simulink model "Linear_Bicycle_Model"  (R2020a)
settings: Solver=VariableStepAuto  StartTime=0.0  StopTime=10  RelTol=1e-3
values from neighbouring files (symbols this model uses):
  c_alpha_f = 156000    [init.m]
  c_alpha_r = 193000    [init.m]
  delta_max = deg2rad(37.3)    [init.m]
  Iz = 2937    [init.m]
  lf = 1.04    [init.m]
  lr = 1.40    (= 1.4)    [init.m]
  mass = 1919    [init.m]
  psi0 = 0*pi/180    (= 0)    [init.m]
  psid0 = 0    [init.m]
  steering_constant = deg2rad(10)    [init.m]
  steering_input_switch = 3    [init.m]
  steering_omega = 0.25    [init.m]
  steering_rate = deg2rad(2)    [init.m]
  v_lat0 = 0    [init.m]
  v_lon0 = 5    [init.m]
  x0 = 0    [init.m]
  y0 = -0.1    [init.m]
libraries: simulink x2
settings Model: Creator=Sameed Quais  LastModifiedBy=Sameed Quais

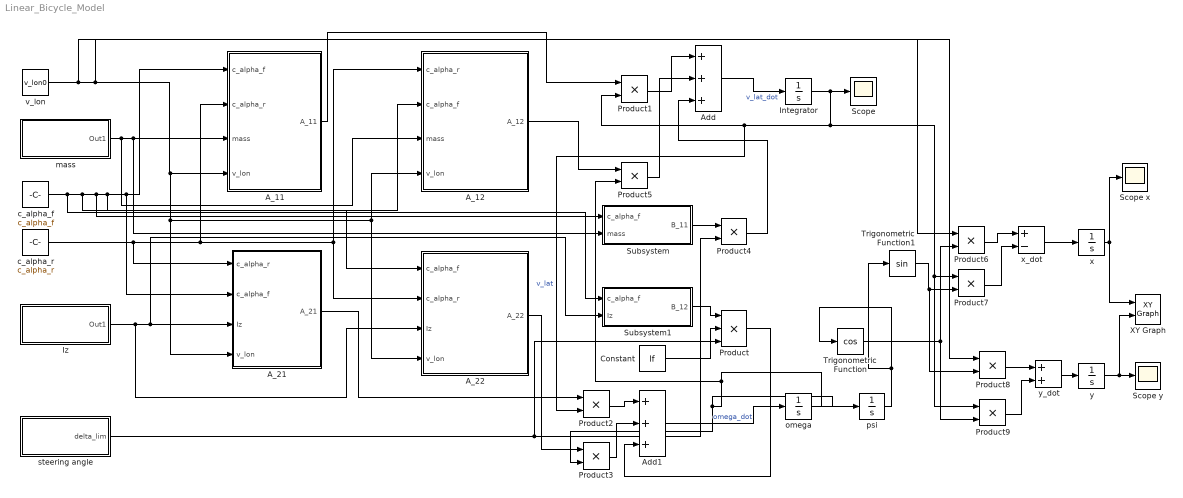
== system Linear_Bicycle_Model ==
  A_11 : Subsystem
  A_12 : Subsystem
  A_21 : Subsystem
  A_22 : Subsystem
  Add : Sum  Inputs=+++
  Add1 : Sum  Inputs=+++
  Constant : Constant  Value=lf
  Integrator : Integrator  InitialCondition=v_lat0
  Iz : Subsystem
  Product : Product  Inputs=3
  Product{1..9} (9 alike) : Product
  Scope : Scope
  Scope x : Scope
  Scope y : Scope
  Subsystem : Subsystem
  Subsystem1 : Subsystem
  Trigonometric Function : Trigonometry  Operator=cos
  Trigonometric Function1 : Trigonometry
  XY Graph : simulink/Sinks/XY Graph  xmin=-inf  xmax=inf  ymin=-inf  ymax=inf  st=-1
  c_alpha_f : Constant  Value=c_alpha_f
  c_alpha_r : Constant  Value=c_alpha_r
  mass : Subsystem
  omega : Integrator  InitialCondition=psi0
  psi : Integrator  InitialCondition=psid0
  steering angle : Subsystem
  v_lon : Constant  Value=v_lon0
  x : Integrator  InitialCondition=x0
  x_dot : Sum  Inputs=+-
  y : Integrator  InitialCondition=y0
  y_dot : Sum
  wires:
  Subsystem1/1(B_12) -> Product/1
  Constant/1 -> Product/2
  mass/1(Out1) -> A_12/3(mass), Subsystem/2(mass), A_11/3(mass)
  v_lon/1 -> Product6/1, Product8/1, A_22/4(v_lon), A_12/4(v_lon), A_21/4(v_lon), A_11/4(v_lon)
  c_alpha_f/1 -> Subsystem1/1(c_alpha_f), A_22/1(c_alpha_f), Subsystem/1(c_alpha_f), A_12/2(c_alpha_f), A_21/2(c_alpha_f), A_11/1(c_alpha_f)
  c_alpha_r/1 -> A_22/2(c_alpha_r), A_12/1(c_alpha_r), A_11/2(c_alpha_r), A_21/1(c_alpha_r)
  Iz/1(Out1) -> A_22/3(Iz), Subsystem1/2(Iz), A_21/3(Iz)
  A_11/1(A_11) -> Product1/1
  Integrator/1 -> Product9/1, Product7/1, Product2/2, Product1/2, Scope/1  "v_lat"
  A_21/1(A_21) -> Product2/1
  omega/1 -> Product3/2, psi/1, Product5/2
  A_22/1(A_22) -> Product3/1
  Subsystem/1(B_11) -> Product4/1
  steering angle/1(delta_lim) -> Product/3, Product4/2
  Product1/1 -> Add/1
  Add/1 -> Integrator/1  "v_lat_dot"
  A_12/1(A_12) -> Product5/1
  Product5/1 -> Add/2
  Product4/1 -> Add/3
  Product2/1 -> Add1/1
  Add1/1 -> omega/1  "omega_dot"
  Product/1 -> Add1/3
  Product3/1 -> Add1/2
  psi/1 -> Trigonometric Function1/1, Trigonometric Function/1
  Trigonometric Function/1 -> Product9/2, Product6/2
  Product6/1 -> x_dot/1
  Trigonometric Function1/1 -> Product8/2, Product7/2
  Product7/1 -> x_dot/2
  x_dot/1 -> x/1
  Product8/1 -> y_dot/1
  Product9/1 -> y_dot/2
  y_dot/1 -> y/1
  x/1 -> Scope x/1, XY Graph/1
  y/1 -> XY Graph/2, Scope y/1

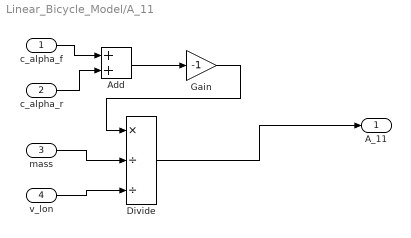
== system Linear_Bicycle_Model/A_11 ==
  c_alpha_f : Inport
  c_alpha_r : Inport  Port=2
  mass : Inport  Port=3
  v_lon : Inport  Port=4
  Add : Sum
  Divide : Product  Inputs=*//
  Gain : Gain  Gain=-1
  A_11 : Outport
  wires:
  c_alpha_r/1 -> Add/2
  c_alpha_f/1 -> Add/1
  mass/1 -> Divide/2
  v_lon/1 -> Divide/3
  Add/1 -> Gain/1
  Gain/1 -> Divide/1
  Divide/1 -> A_11/1

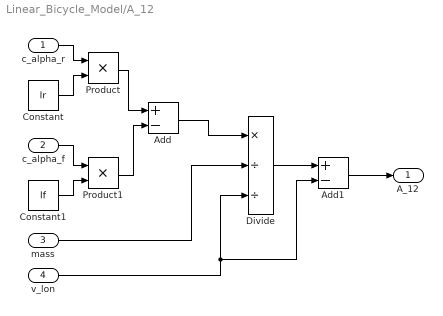
== system Linear_Bicycle_Model/A_12 ==
  c_alpha_r : Inport
  c_alpha_f : Inport  Port=2
  mass : Inport  Port=3
  v_lon : Inport  Port=4
  Add : Sum  Inputs=+-
  Add1 : Sum  Inputs=+-
  Constant : Constant  Value=lr
  Constant1 : Constant  Value=lf
  Divide : Product  Inputs=*//
  Product : Product
  Product1 : Product
  A_12 : Outport
  wires:
  c_alpha_r/1 -> Product/1
  Constant/1 -> Product/2
  c_alpha_f/1 -> Product1/1
  Constant1/1 -> Product1/2
  Product/1 -> Add/1
  Product1/1 -> Add/2
  Add/1 -> Divide/1
  mass/1 -> Divide/2
  v_lon/1 -> Add1/2, Divide/3
  Divide/1 -> Add1/1
  Add1/1 -> A_12/1

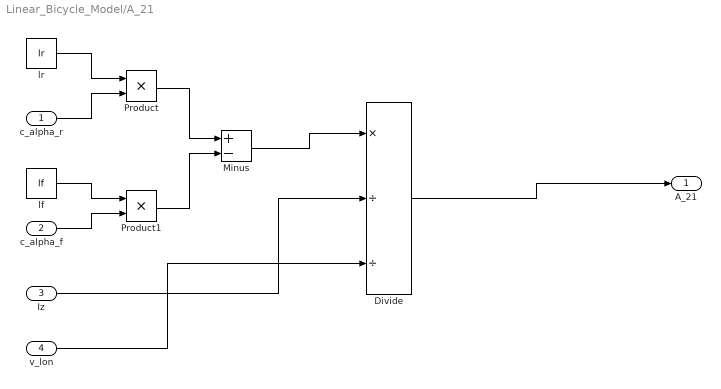
== system Linear_Bicycle_Model/A_21 ==
  c_alpha_r : Inport
  c_alpha_f : Inport  Port=2
  Iz : Inport  Port=3
  v_lon : Inport  Port=4
  Divide : Product  Inputs=*//
  Minus : Sum  Inputs=+-
  Product : Product
  Product1 : Product
  lf : Constant  Value=lf
  lr : Constant  Value=lr
  A_21 : Outport
  wires:
  lr/1 -> Product/1
  c_alpha_r/1 -> Product/2
  lf/1 -> Product1/1
  c_alpha_f/1 -> Product1/2
  Product/1 -> Minus/1
  Product1/1 -> Minus/2
  Minus/1 -> Divide/1
  Iz/1 -> Divide/2
  v_lon/1 -> Divide/3
  Divide/1 -> A_21/1

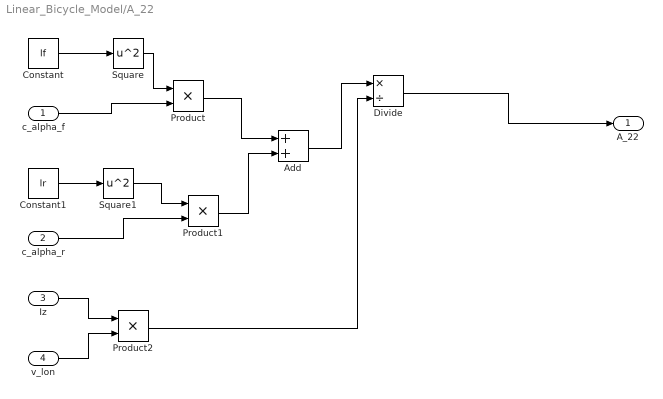
== system Linear_Bicycle_Model/A_22 ==
  c_alpha_f : Inport
  c_alpha_r : Inport  Port=2
  Iz : Inport  Port=3
  v_lon : Inport  Port=4
  Add : Sum
  Constant : Constant  Value=lf
  Constant1 : Constant  Value=lr
  Divide : Product  Inputs=*/
  Product : Product
  Product1 : Product
  Product2 : Product
  Square : Math  Operator=square  SaturateOnIntegerOverflow=on
  Square1 : Math  Operator=square  SaturateOnIntegerOverflow=on
  A_22 : Outport
  wires:
  Constant/1 -> Square/1
  Square/1 -> Product/1
  c_alpha_f/1 -> Product/2
  Constant1/1 -> Square1/1
  c_alpha_r/1 -> Product1/2
  Square1/1 -> Product1/1
  Product/1 -> Add/1
  Product1/1 -> Add/2
  Add/1 -> Divide/1
  Iz/1 -> Product2/1
  v_lon/1 -> Product2/2
  Product2/1 -> Divide/2
  Divide/1 -> A_22/1

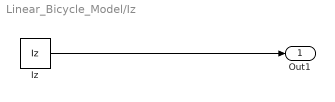
== system Linear_Bicycle_Model/Iz ==
  Iz : Constant  Value=Iz
  Out1 : Outport
  wires:
  Iz/1 -> Out1/1

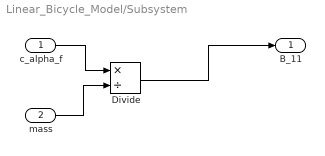
== system Linear_Bicycle_Model/Subsystem ==
  c_alpha_f : Inport
  mass : Inport  Port=2
  Divide : Product  Inputs=*/
  B_11 : Outport
  wires:
  c_alpha_f/1 -> Divide/1
  mass/1 -> Divide/2
  Divide/1 -> B_11/1

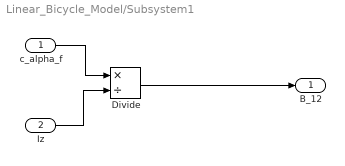
== system Linear_Bicycle_Model/Subsystem1 ==
  c_alpha_f : Inport
  Iz : Inport  Port=2
  Divide : Product  Inputs=*/
  B_12 : Outport
  wires:
  c_alpha_f/1 -> Divide/1
  Iz/1 -> Divide/2
  Divide/1 -> B_12/1

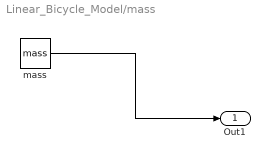
== system Linear_Bicycle_Model/mass ==
  mass : Constant  Value=mass
  Out1 : Outport
  wires:
  mass/1 -> Out1/1

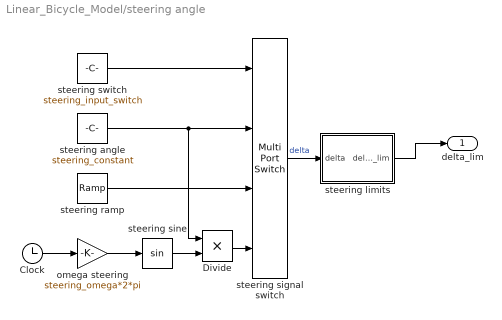
== system Linear_Bicycle_Model/steering angle ==
  Clock : Clock
  Divide : Product
  omega steering : Gain  Gain=steering_omega*2*pi
  steering angle : Constant  Value=steering_constant
  steering limits : Subsystem
  steering ramp : simulink/Sources/Ramp  slope=steering_rate  start=0  InitialOutput=0
  steering sine : Trigonometry
  steering switch : Constant  Value=steering_input_switch
  steering signal switch : MultiPortSwitch
  delta_lim : Outport
  wires:
  steering signal switch/1 -> steering limits/1(delta)  "delta"
  Clock/1 -> omega steering/1
  Divide/1 -> steering signal switch/4
  steering sine/1 -> Divide/2
  steering ramp/1 -> steering signal switch/3
  omega steering/1 -> steering sine/1
  steering angle/1 -> Divide/1, steering signal switch/2
  steering switch/1 -> steering signal switch/1
  steering limits/1(delta_lim) -> delta_lim/1

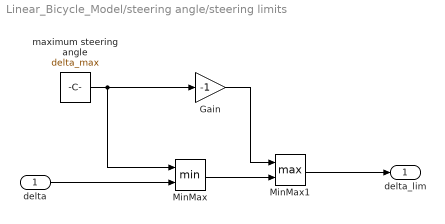
== system Linear_Bicycle_Model/steering angle/steering limits ==
  delta : Inport
  Gain : Gain  Gain=-1
  MinMax : MinMax  Inputs=2
  MinMax1 : MinMax  Function=max  Inputs=2
  maximum steering angle : Constant  Value=delta_max
  delta_lim : Outport  VectorParamsAs1DForOutWhenUnconnected=off
  wires:
  MinMax1/1 -> delta_lim/1
  delta/1 -> MinMax/2
  maximum steering angle/1 -> Gain/1, MinMax/1
  MinMax/1 -> MinMax1/2
  Gain/1 -> MinMax1/1
